simulink model "compare_filters"  (R2025a)
settings: Solver=VariableStepAuto  StartTime=0.0  StopTime=1.5  RelTol=1e-3
values from neighbouring files (symbols this model uses):
  phi_corr_LUT_param = Simulink.Parameter(phi_corr_LUT)    [lut_script.m]
undefined symbols (not defined in the file or in its folder): closed_loop, D_duty_cycle, D_m, DiscIntNeverNeededParam, hall_errors, I_duty_cycle, J_t, L_ss, lambda_m, P, P_duty_cycle, r_s, R_vs, T_m, theta_v, use_LUT, V_bus
libraries: spsMosfetLib x18, spsSeriesRLCBranchLib x12, spsVoltageMeasurementLib x9, spsControlledCurrentSourceLib x9, slpidlib x6, eeGeneralControl x3, simulink x3, embmathops x3, spsControlledVoltageSourceLib x3, spsPWMGeneratorDCDCLib x3, spsDCVoltageSourceLib x3, sps_lib x3
(part 3 of 3)

== system compare_filters/3_phase/hall_filter/hardware_ISR_routine/Subsystem1 ==
  In1 : Inport
  Memory{,1..5} (6 alike) : Memory  InheritSampleTime=on
  Mux : Mux  Inputs=6
  Sum{,1..5} (6 alike) : Sum  Inputs=|+-
  tau_vec : Outport
  wires:
  Memory1/1 -> Sum1/2, Sum2/1, Memory2/1
  Memory/1 -> Sum1/1, Sum/2, Memory1/1
  Memory2/1 -> Sum3/1, Sum2/2, Memory3/1
  In1/1 -> Sum/1, Memory/1
  Memory3/1 -> Sum4/1, Sum3/2, Memory4/1
  Memory4/1 -> Memory5/1, Sum5/1, Sum4/2
  Mux/1 -> tau_vec/1
  Memory5/1 -> Sum5/2
  Sum/1 -> Mux/1
  Sum1/1 -> Mux/2
  Sum2/1 -> Mux/3
  Sum3/1 -> Mux/4
  Sum4/1 -> Mux/5
  Sum5/1 -> Mux/6

== system compare_filters/3_phase/hall_filter/hardware_ISR_routine/Subsystem2 ==
  timer : Inport
  Data Store Write2 : DataStoreWrite  DataStoreName=t_now  IndexOptions=Index vector (dialog)  Indices=1  OutputSizes=1
  wires:
  timer/1 -> Data Store Write2/1

== system compare_filters/3_phase/hall_filter/hardware_ISR_routine/Subsystem3 ==
  tau_now_write : Inport
  tau_next_write : Inport  Port=2
  update_now : Inport  Port=3
  update_next : Inport  Port=4
  Enable : EnablePort
  Subsystem : Subsystem
  Subsystem1 : Subsystem
  wires:
  tau_now_write/1 -> Subsystem/1(tau_now_write)
  tau_next_write/1 -> Subsystem1/1(tau_next_write)
  update_now/1 -> Subsystem/Enable
  update_next/1 -> Subsystem1/Enable

== system compare_filters/3_phase/hall_filter/software_ISR_routine/Subsystem ==
  Data Store Read : DataStoreRead  DataStoreName=tau_corr_next  IndexOptions=Index vector (dialog)  Indices=1  OutputSizes=1
  Data Store Write : DataStoreWrite  DataStoreName=tau_corr_now  IndexOptions=Index vector (dialog)  Indices=1  OutputSizes=1
  wires:
  Data Store Read/1 -> Data Store Write/1

== system compare_filters/3_phase/hall_filter/software_ISR_routine/Subsystem1 ==
  Constant : Constant  Value=-1
  Data Store Write1 : DataStoreWrite  DataStoreName=tau_corr_next  IndexOptions=Index vector (dialog)  Indices=1  OutputSizes=1
  wires:
  Constant/1 -> Data Store Write1/1

== system compare_filters/3_phase/hall_filter/software_ISR_routine/Subsystem2 ==
  Constant : Constant
  Data Store Read : DataStoreRead  DataStoreName=state_out  IndexOptions=Index vector (dialog)  Indices=1  OutputSizes=1
  Data Store Write : DataStoreWrite  DataStoreName=state_out  IndexOptions=Index vector (dialog)  Indices=1  OutputSizes=1
  Modulo by Constant : embmathops/Modulo by Constant  Denominator=6  SimulateUsing=Code generation
  Sum : Sum  Inputs=|++
  wires:
  Constant/1 -> Sum/2
  Data Store Read/1 -> Sum/1
  Sum/1 -> Modulo by Constant/1
  Modulo by Constant/1 -> Data Store Write/1

== system compare_filters/3_phase/hall_filter/software_ISR_routine/Subsystem3 ==
  Constant : Constant
  Data Store Read : DataStoreRead  DataStoreName=state_out  IndexOptions=Index vector (dialog)  Indices=1  OutputSizes=1
  Sum : Sum  Inputs=|++
  state_out : Outport
  wires:
  Data Store Read/1 -> Sum/1
  Sum/1 -> state_out/1
  Constant/1 -> Sum/2

== system compare_filters/3_phase/hall_filter/software_ISR_routine/Subsystem4 ==
  Constant : Constant  Value=0
  Data Store Write : DataStoreWrite  DataStoreName=first_time  IndexOptions=Index vector (dialog)  Indices=1  OutputSizes=1
  wires:
  Constant/1 -> Data Store Write/1

== system compare_filters/from_LUT/hall_filter/calibration_routine/Subsystem ==
  Constant : Constant  Value=pi/3
  Data Store Read : DataStoreRead  DataStoreName=tau_corr_now  IndexOptions=Index vector (dialog)  Indices=1  OutputSizes=1
  Data Store Write : DataStoreWrite  DataStoreName=omega_now  IndexOptions=Index vector (dialog)  Indices=1  OutputSizes=1
  Divide : Product  Inputs=*/
  wires:
  Data Store Read/1 -> Divide/2
  Constant/1 -> Divide/1
  Divide/1 -> Data Store Write/1

== system compare_filters/from_LUT/hall_filter/calibration_routine/Subsystem1 ==
  Data Store Read : DataStoreRead  DataStoreName=tau_corr_now  IndexOptions=Index vector (dialog)  Indices=1  OutputSizes=1
  Data Store Read1 : DataStoreRead  DataStoreName=omega_now  IndexOptions=Index vector (dialog)  Indices=1  OutputSizes=1
  Data Store Write : DataStoreWrite  DataStoreName=del_phi  IndexOptions=Index vector (dialog)  Indices=1  OutputSizes=1
  Product : Product
  wires:
  Data Store Read/1 -> Product/1
  Data Store Read1/1 -> Product/2
  Product/1 -> Data Store Write/1

== system compare_filters/from_LUT/hall_filter/calibration_routine/Subsystem2 ==
  Constant : Constant  Value=6
  Constant1 : Constant  Value=0.02
  Constant2 : Constant  Value=4e-4
  Constant3 : Constant  Value=50
  Data Store Read1 : DataStoreRead  DataStoreName=state_out  IndexOptions=Index vector (dialog)  Indices=1  OutputSizes=1
  Data Store Read2 : DataStoreRead  DataStoreName=del_phi  IndexOptions=Index vector (dialog)  Indices=1  OutputSizes=1
  Data Store Read3 : DataStoreRead  DataStoreName=LUT_phi  IndexOptions=Index vector (dialog)  Indices=1  OutputSizes=1
  Data Store Read4 : DataStoreRead  DataStoreName=LUT_var  IndexOptions=Index vector (dialog)  Indices=1  OutputSizes=1
  Data Store Read5 : DataStoreRead  DataStoreName=LUT_count  IndexOptions=Index vector (dialog)  Indices=1  OutputSizes=1
  Data Store Read6 : DataStoreRead  DataStoreName=LUT_valid  IndexOptions=Index vector (dialog)  Indices=1  OutputSizes=1
  Data Store Read7 : DataStoreRead  DataStoreName=cal_done  IndexOptions=Index vector (dialog)  Indices=1  OutputSizes=1
  Data Store Write : DataStoreWrite  DataStoreName=LUT_phi  IndexOptions=Index vector (dialog)  Indices=1  OutputSizes=1
  Data Store Write1 : DataStoreWrite  DataStoreName=LUT_var  IndexOptions=Index vector (dialog)  Indices=1  OutputSizes=1
  Data Store Write2 : DataStoreWrite  DataStoreName=LUT_count  IndexOptions=Index vector (dialog)  Indices=1  OutputSizes=1
  Data Store Write3 : DataStoreWrite  DataStoreName=LUT_valid  IndexOptions=Index vector (dialog)  Indices=1  OutputSizes=1
  Data Store Write4 : DataStoreWrite  DataStoreName=cal_done  IndexOptions=Index vector (dialog)  Indices=1  OutputSizes=1
  MATLAB Function : MATLAB Function  TreatAsAtomicUnit=on
  wires:
  Data Store Read1/1 -> MATLAB Function/1(k)
  Data Store Read2/1 -> MATLAB Function/2(dphi)
  Data Store Read3/1 -> MATLAB Function/3(phi)
  Data Store Read4/1 -> MATLAB Function/4(varv)
  Data Store Read5/1 -> MATLAB Function/5(cnt)
  Data Store Read6/1 -> MATLAB Function/6(valid)
  Data Store Read7/1 -> MATLAB Function/7(done)
  Constant/1 -> MATLAB Function/8(Nsteady)
  Constant1/1 -> MATLAB Function/9(deadband_rad)
  Constant2/1 -> MATLAB Function/10(var_max)
  Constant3/1 -> MATLAB Function/11(omega_min)
  MATLAB Function/1(phi_n) -> Data Store Write/1
  MATLAB Function/2(varv_n) -> Data Store Write1/1
  MATLAB Function/3(cnt_n) -> Data Store Write2/1
  MATLAB Function/4(valid_n) -> Data Store Write3/1
  MATLAB Function/5(done_n) -> Data Store Write4/1

== system compare_filters/from_LUT/hall_filter/hardware_ISR_routine/Atomic Subsystem ==
  tau_now_write : Inport
  tau_next_write : Inport  Port=2
  update_now : Inport  Port=3
  update_next : Inport  Port=4
  software_ISR_enable : EnablePort
  Subsystem : Subsystem
  Subsystem1 : Subsystem
  wires:
  tau_next_write/1 -> Subsystem1/1(tau_next_write)
  update_now/1 -> Subsystem/Enable
  update_next/1 -> Subsystem1/Enable
  tau_now_write/1 -> Subsystem/1(tau_now_write)

== system compare_filters/from_LUT/hall_filter/hardware_ISR_routine/Subsystem ==
  Constant : Constant
  Data Store Read : DataStoreRead  DataStoreName=reset_toggle  IndexOptions=Index vector (dialog)  Indices=1  OutputSizes=1
  Data Store Read1 : DataStoreRead  DataStoreName=time_base  IndexOptions=Index vector (dialog)  Indices=1  OutputSizes=1
  Data Store Read2 : DataStoreRead  DataStoreName=t_now  IndexOptions=Index vector (dialog)  Indices=1  OutputSizes=1
  Data Store Write : DataStoreWrite  DataStoreName=reset_toggle  IndexOptions=Index vector (dialog)  Indices=1  OutputSizes=1
  Data Store Write1 : DataStoreWrite  DataStoreName=time_base  IndexOptions=Index vector (dialog)  Indices=1  OutputSizes=1
  Sum : Sum  Inputs=|-+
  Sum1 : Sum  Inputs=|++
  wires:
  Sum/1 -> Data Store Write/1  "reset_val"
  Data Store Read/1 -> Sum/1
  Constant/1 -> Sum/2
  Data Store Read1/1 -> Sum1/1
  Sum1/1 -> Data Store Write1/1
  Data Store Read2/1 -> Sum1/2

== system compare_filters/from_LUT/hall_filter/hardware_ISR_routine/Subsystem1 ==
  In1 : Inport
  Memory{,1..5} (6 alike) : Memory  InheritSampleTime=on
  Mux : Mux  Inputs=6
  Sum{,1..5} (6 alike) : Sum  Inputs=|+-
  tau_vec : Outport
  wires:
  Memory1/1 -> Sum1/2, Sum2/1, Memory2/1
  Memory/1 -> Sum1/1, Sum/2, Memory1/1
  Memory2/1 -> Sum3/1, Sum2/2, Memory3/1
  In1/1 -> Sum/1, Memory/1
  Memory3/1 -> Sum4/1, Sum3/2, Memory4/1
  Memory4/1 -> Memory5/1, Sum5/1, Sum4/2
  Mux/1 -> tau_vec/1
  Memory5/1 -> Sum5/2
  Sum/1 -> Mux/1
  Sum1/1 -> Mux/2
  Sum2/1 -> Mux/3
  Sum3/1 -> Mux/4
  Sum4/1 -> Mux/5
  Sum5/1 -> Mux/6

== system compare_filters/from_LUT/hall_filter/hardware_ISR_routine/Subsystem2 ==
  timer : Inport
  Data Store Write2 : DataStoreWrite  DataStoreName=t_now  IndexOptions=Index vector (dialog)  Indices=1  OutputSizes=1
  wires:
  timer/1 -> Data Store Write2/1

== system compare_filters/from_LUT/hall_filter/hardware_ISR_routine/Subsystem3 ==
  tau_now_write : Inport
  tau_next_write : Inport  Port=2
  update_now : Inport  Port=3
  update_next : Inport  Port=4
  Enable : EnablePort
  Subsystem : Subsystem
  Subsystem1 : Subsystem
  wires:
  tau_now_write/1 -> Subsystem/1(tau_now_write)
  tau_next_write/1 -> Subsystem1/1(tau_next_write)
  update_now/1 -> Subsystem/Enable
  update_next/1 -> Subsystem1/Enable

== system compare_filters/from_LUT/hall_filter/software_ISR_routine/Subsystem ==
  Data Store Read : DataStoreRead  DataStoreName=tau_corr_next  IndexOptions=Index vector (dialog)  Indices=1  OutputSizes=1
  Data Store Write : DataStoreWrite  DataStoreName=tau_corr_now  IndexOptions=Index vector (dialog)  Indices=1  OutputSizes=1
  wires:
  Data Store Read/1 -> Data Store Write/1

== system compare_filters/from_LUT/hall_filter/software_ISR_routine/Subsystem1 ==
  Constant : Constant  Value=-1
  Data Store Write1 : DataStoreWrite  DataStoreName=tau_corr_next  IndexOptions=Index vector (dialog)  Indices=1  OutputSizes=1
  wires:
  Constant/1 -> Data Store Write1/1

== system compare_filters/from_LUT/hall_filter/software_ISR_routine/Subsystem2 ==
  Constant : Constant
  Data Store Read : DataStoreRead  DataStoreName=state_out  IndexOptions=Index vector (dialog)  Indices=1  OutputSizes=1
  Data Store Write : DataStoreWrite  DataStoreName=state_out  IndexOptions=Index vector (dialog)  Indices=1  OutputSizes=1
  Modulo by Constant : embmathops/Modulo by Constant  Denominator=6  SimulateUsing=Code generation
  Sum : Sum  Inputs=|++
  wires:
  Constant/1 -> Sum/2
  Data Store Read/1 -> Sum/1
  Sum/1 -> Modulo by Constant/1
  Modulo by Constant/1 -> Data Store Write/1

== system compare_filters/from_LUT/hall_filter/software_ISR_routine/Subsystem3 ==
  Constant : Constant
  Data Store Read : DataStoreRead  DataStoreName=state_out  IndexOptions=Index vector (dialog)  Indices=1  OutputSizes=1
  Sum : Sum  Inputs=|++
  state_out : Outport
  wires:
  Data Store Read/1 -> Sum/1
  Sum/1 -> state_out/1
  Constant/1 -> Sum/2

== system compare_filters/from_LUT/hall_filter/software_ISR_routine/Subsystem4 ==
  Constant : Constant  Value=0
  Data Store Write : DataStoreWrite  DataStoreName=first_time  IndexOptions=Index vector (dialog)  Indices=1  OutputSizes=1
  wires:
  Constant/1 -> Data Store Write/1

== system compare_filters/no_LUT/hall_filter/calibration_routine/Subsystem ==
  Constant : Constant  Value=pi/3
  Data Store Read : DataStoreRead  DataStoreName=tau_corr_now  IndexOptions=Index vector (dialog)  Indices=1  OutputSizes=1
  Data Store Write : DataStoreWrite  DataStoreName=omega_now  IndexOptions=Index vector (dialog)  Indices=1  OutputSizes=1
  Divide : Product  Inputs=*/
  wires:
  Data Store Read/1 -> Divide/2
  Constant/1 -> Divide/1
  Divide/1 -> Data Store Write/1

== system compare_filters/no_LUT/hall_filter/calibration_routine/Subsystem1 ==
  Data Store Read : DataStoreRead  DataStoreName=tau_corr_now  IndexOptions=Index vector (dialog)  Indices=1  OutputSizes=1
  Data Store Read1 : DataStoreRead  DataStoreName=omega_now  IndexOptions=Index vector (dialog)  Indices=1  OutputSizes=1
  Data Store Write : DataStoreWrite  DataStoreName=del_phi  IndexOptions=Index vector (dialog)  Indices=1  OutputSizes=1
  Product : Product
  wires:
  Data Store Read/1 -> Product/1
  Data Store Read1/1 -> Product/2
  Product/1 -> Data Store Write/1

== system compare_filters/no_LUT/hall_filter/calibration_routine/Subsystem2 ==
  Constant : Constant  Value=6
  Constant1 : Constant  Value=0.02
  Constant2 : Constant  Value=4e-4
  Constant3 : Constant  Value=50
  Data Store Read1 : DataStoreRead  DataStoreName=state_out  IndexOptions=Index vector (dialog)  Indices=1  OutputSizes=1
  Data Store Read2 : DataStoreRead  DataStoreName=del_phi  IndexOptions=Index vector (dialog)  Indices=1  OutputSizes=1
  Data Store Read3 : DataStoreRead  DataStoreName=LUT_phi  IndexOptions=Index vector (dialog)  Indices=1  OutputSizes=1
  Data Store Read4 : DataStoreRead  DataStoreName=LUT_var  IndexOptions=Index vector (dialog)  Indices=1  OutputSizes=1
  Data Store Read5 : DataStoreRead  DataStoreName=LUT_count  IndexOptions=Index vector (dialog)  Indices=1  OutputSizes=1
  Data Store Read6 : DataStoreRead  DataStoreName=LUT_valid  IndexOptions=Index vector (dialog)  Indices=1  OutputSizes=1
  Data Store Read7 : DataStoreRead  DataStoreName=cal_done  IndexOptions=Index vector (dialog)  Indices=1  OutputSizes=1
  Data Store Write : DataStoreWrite  DataStoreName=LUT_phi  IndexOptions=Index vector (dialog)  Indices=1  OutputSizes=1
  Data Store Write1 : DataStoreWrite  DataStoreName=LUT_var  IndexOptions=Index vector (dialog)  Indices=1  OutputSizes=1
  Data Store Write2 : DataStoreWrite  DataStoreName=LUT_count  IndexOptions=Index vector (dialog)  Indices=1  OutputSizes=1
  Data Store Write3 : DataStoreWrite  DataStoreName=LUT_valid  IndexOptions=Index vector (dialog)  Indices=1  OutputSizes=1
  Data Store Write4 : DataStoreWrite  DataStoreName=cal_done  IndexOptions=Index vector (dialog)  Indices=1  OutputSizes=1
  MATLAB Function : MATLAB Function  TreatAsAtomicUnit=on
  wires:
  Data Store Read1/1 -> MATLAB Function/1(k)
  Data Store Read2/1 -> MATLAB Function/2(dphi)
  Data Store Read3/1 -> MATLAB Function/3(phi)
  Data Store Read4/1 -> MATLAB Function/4(varv)
  Data Store Read5/1 -> MATLAB Function/5(cnt)
  Data Store Read6/1 -> MATLAB Function/6(valid)
  Data Store Read7/1 -> MATLAB Function/7(done)
  Constant/1 -> MATLAB Function/8(Nsteady)
  Constant1/1 -> MATLAB Function/9(deadband_rad)
  Constant2/1 -> MATLAB Function/10(var_max)
  Constant3/1 -> MATLAB Function/11(omega_min)
  MATLAB Function/1(phi_n) -> Data Store Write/1
  MATLAB Function/2(varv_n) -> Data Store Write1/1
  MATLAB Function/3(cnt_n) -> Data Store Write2/1
  MATLAB Function/4(valid_n) -> Data Store Write3/1
  MATLAB Function/5(done_n) -> Data Store Write4/1

== system compare_filters/no_LUT/hall_filter/hardware_ISR_routine/Atomic Subsystem ==
  tau_now_write : Inport
  tau_next_write : Inport  Port=2
  update_now : Inport  Port=3
  update_next : Inport  Port=4
  software_ISR_enable : EnablePort
  Subsystem : Subsystem
  Subsystem1 : Subsystem
  wires:
  tau_next_write/1 -> Subsystem1/1(tau_next_write)
  update_now/1 -> Subsystem/Enable
  update_next/1 -> Subsystem1/Enable
  tau_now_write/1 -> Subsystem/1(tau_now_write)

== system compare_filters/no_LUT/hall_filter/hardware_ISR_routine/Subsystem ==
  Constant : Constant
  Data Store Read : DataStoreRead  DataStoreName=reset_toggle  IndexOptions=Index vector (dialog)  Indices=1  OutputSizes=1
  Data Store Read1 : DataStoreRead  DataStoreName=time_base  IndexOptions=Index vector (dialog)  Indices=1  OutputSizes=1
  Data Store Read2 : DataStoreRead  DataStoreName=t_now  IndexOptions=Index vector (dialog)  Indices=1  OutputSizes=1
  Data Store Write : DataStoreWrite  DataStoreName=reset_toggle  IndexOptions=Index vector (dialog)  Indices=1  OutputSizes=1
  Data Store Write1 : DataStoreWrite  DataStoreName=time_base  IndexOptions=Index vector (dialog)  Indices=1  OutputSizes=1
  Sum : Sum  Inputs=|-+
  Sum1 : Sum  Inputs=|++
  wires:
  Sum/1 -> Data Store Write/1  "reset_val"
  Data Store Read/1 -> Sum/1
  Constant/1 -> Sum/2
  Data Store Read1/1 -> Sum1/1
  Sum1/1 -> Data Store Write1/1
  Data Store Read2/1 -> Sum1/2

== system compare_filters/no_LUT/hall_filter/hardware_ISR_routine/Subsystem1 ==
  In1 : Inport
  Memory{,1..5} (6 alike) : Memory  InheritSampleTime=on
  Mux : Mux  Inputs=6
  Sum{,1..5} (6 alike) : Sum  Inputs=|+-
  tau_vec : Outport
  wires:
  Memory1/1 -> Sum1/2, Sum2/1, Memory2/1
  Memory/1 -> Sum1/1, Sum/2, Memory1/1
  Memory2/1 -> Sum3/1, Sum2/2, Memory3/1
  In1/1 -> Sum/1, Memory/1
  Memory3/1 -> Sum4/1, Sum3/2, Memory4/1
  Memory4/1 -> Memory5/1, Sum5/1, Sum4/2
  Mux/1 -> tau_vec/1
  Memory5/1 -> Sum5/2
  Sum/1 -> Mux/1
  Sum1/1 -> Mux/2
  Sum2/1 -> Mux/3
  Sum3/1 -> Mux/4
  Sum4/1 -> Mux/5
  Sum5/1 -> Mux/6

== system compare_filters/no_LUT/hall_filter/hardware_ISR_routine/Subsystem2 ==
  timer : Inport
  Data Store Write2 : DataStoreWrite  DataStoreName=t_now  IndexOptions=Index vector (dialog)  Indices=1  OutputSizes=1
  wires:
  timer/1 -> Data Store Write2/1

== system compare_filters/no_LUT/hall_filter/hardware_ISR_routine/Subsystem3 ==
  tau_now_write : Inport
  tau_next_write : Inport  Port=2
  update_now : Inport  Port=3
  update_next : Inport  Port=4
  Enable : EnablePort
  Subsystem : Subsystem
  Subsystem1 : Subsystem
  wires:
  tau_now_write/1 -> Subsystem/1(tau_now_write)
  tau_next_write/1 -> Subsystem1/1(tau_next_write)
  update_now/1 -> Subsystem/Enable
  update_next/1 -> Subsystem1/Enable

== system compare_filters/no_LUT/hall_filter/software_ISR_routine/Subsystem ==
  Data Store Read : DataStoreRead  DataStoreName=tau_corr_next  IndexOptions=Index vector (dialog)  Indices=1  OutputSizes=1
  Data Store Write : DataStoreWrite  DataStoreName=tau_corr_now  IndexOptions=Index vector (dialog)  Indices=1  OutputSizes=1
  wires:
  Data Store Read/1 -> Data Store Write/1

== system compare_filters/no_LUT/hall_filter/software_ISR_routine/Subsystem1 ==
  Constant : Constant  Value=-1
  Data Store Write1 : DataStoreWrite  DataStoreName=tau_corr_next  IndexOptions=Index vector (dialog)  Indices=1  OutputSizes=1
  wires:
  Constant/1 -> Data Store Write1/1

== system compare_filters/no_LUT/hall_filter/software_ISR_routine/Subsystem2 ==
  Constant : Constant
  Data Store Read : DataStoreRead  DataStoreName=state_out  IndexOptions=Index vector (dialog)  Indices=1  OutputSizes=1
  Data Store Write : DataStoreWrite  DataStoreName=state_out  IndexOptions=Index vector (dialog)  Indices=1  OutputSizes=1
  Modulo by Constant : embmathops/Modulo by Constant  Denominator=6  SimulateUsing=Code generation
  Sum : Sum  Inputs=|++
  wires:
  Constant/1 -> Sum/2
  Data Store Read/1 -> Sum/1
  Sum/1 -> Modulo by Constant/1
  Modulo by Constant/1 -> Data Store Write/1

== system compare_filters/no_LUT/hall_filter/software_ISR_routine/Subsystem3 ==
  Constant : Constant
  Data Store Read : DataStoreRead  DataStoreName=state_out  IndexOptions=Index vector (dialog)  Indices=1  OutputSizes=1
  Sum : Sum  Inputs=|++
  state_out : Outport
  wires:
  Data Store Read/1 -> Sum/1
  Sum/1 -> state_out/1
  Constant/1 -> Sum/2

== system compare_filters/no_LUT/hall_filter/software_ISR_routine/Subsystem4 ==
  Constant : Constant  Value=0
  Data Store Write : DataStoreWrite  DataStoreName=first_time  IndexOptions=Index vector (dialog)  Indices=1  OutputSizes=1
  wires:
  Constant/1 -> Data Store Write/1

== system compare_filters/3_phase/hall_filter/hardware_ISR_routine/Atomic Subsystem/Subsystem ==
  tau_now_write : Inport
  update_now : EnablePort
  Data Store Write : DataStoreWrite  DataStoreName=tau_corr_now  IndexOptions=Index vector (dialog)  Indices=1  OutputSizes=1
  wires:
  tau_now_write/1 -> Data Store Write/1

== system compare_filters/3_phase/hall_filter/hardware_ISR_routine/Atomic Subsystem/Subsystem1 ==
  tau_next_write : Inport
  update_next : EnablePort
  Data Store Write1 : DataStoreWrite  DataStoreName=tau_corr_next  IndexOptions=Index vector (dialog)  Indices=1  OutputSizes=1
  wires:
  tau_next_write/1 -> Data Store Write1/1

== system compare_filters/3_phase/hall_filter/hardware_ISR_routine/Subsystem3/Subsystem ==
  tau_now_write : Inport
  update_now : EnablePort
  Data Store Write : DataStoreWrite  DataStoreName=tau_corr_now  IndexOptions=Index vector (dialog)  Indices=1  OutputSizes=1
  wires:
  tau_now_write/1 -> Data Store Write/1

== system compare_filters/3_phase/hall_filter/hardware_ISR_routine/Subsystem3/Subsystem1 ==
  tau_next_write : Inport
  update_next : EnablePort
  Data Store Write1 : DataStoreWrite  DataStoreName=tau_corr_next  IndexOptions=Index vector (dialog)  Indices=1  OutputSizes=1
  wires:
  tau_next_write/1 -> Data Store Write1/1

== system compare_filters/from_LUT/hall_filter/hardware_ISR_routine/Atomic Subsystem/Subsystem ==
  tau_now_write : Inport
  update_now : EnablePort
  Data Store Write : DataStoreWrite  DataStoreName=tau_corr_now  IndexOptions=Index vector (dialog)  Indices=1  OutputSizes=1
  wires:
  tau_now_write/1 -> Data Store Write/1

== system compare_filters/from_LUT/hall_filter/hardware_ISR_routine/Atomic Subsystem/Subsystem1 ==
  tau_next_write : Inport
  update_next : EnablePort
  Data Store Write1 : DataStoreWrite  DataStoreName=tau_corr_next  IndexOptions=Index vector (dialog)  Indices=1  OutputSizes=1
  wires:
  tau_next_write/1 -> Data Store Write1/1

== system compare_filters/from_LUT/hall_filter/hardware_ISR_routine/Subsystem3/Subsystem ==
  tau_now_write : Inport
  update_now : EnablePort
  Data Store Write : DataStoreWrite  DataStoreName=tau_corr_now  IndexOptions=Index vector (dialog)  Indices=1  OutputSizes=1
  wires:
  tau_now_write/1 -> Data Store Write/1

== system compare_filters/from_LUT/hall_filter/hardware_ISR_routine/Subsystem3/Subsystem1 ==
  tau_next_write : Inport
  update_next : EnablePort
  Data Store Write1 : DataStoreWrite  DataStoreName=tau_corr_next  IndexOptions=Index vector (dialog)  Indices=1  OutputSizes=1
  wires:
  tau_next_write/1 -> Data Store Write1/1

== system compare_filters/no_LUT/hall_filter/hardware_ISR_routine/Atomic Subsystem/Subsystem ==
  tau_now_write : Inport
  update_now : EnablePort
  Data Store Write : DataStoreWrite  DataStoreName=tau_corr_now  IndexOptions=Index vector (dialog)  Indices=1  OutputSizes=1
  wires:
  tau_now_write/1 -> Data Store Write/1

== system compare_filters/no_LUT/hall_filter/hardware_ISR_routine/Atomic Subsystem/Subsystem1 ==
  tau_next_write : Inport
  update_next : EnablePort
  Data Store Write1 : DataStoreWrite  DataStoreName=tau_corr_next  IndexOptions=Index vector (dialog)  Indices=1  OutputSizes=1
  wires:
  tau_next_write/1 -> Data Store Write1/1

== system compare_filters/no_LUT/hall_filter/hardware_ISR_routine/Subsystem3/Subsystem ==
  tau_now_write : Inport
  update_now : EnablePort
  Data Store Write : DataStoreWrite  DataStoreName=tau_corr_now  IndexOptions=Index vector (dialog)  Indices=1  OutputSizes=1
  wires:
  tau_now_write/1 -> Data Store Write/1

== system compare_filters/no_LUT/hall_filter/hardware_ISR_routine/Subsystem3/Subsystem1 ==
  tau_next_write : Inport
  update_next : EnablePort
  Data Store Write1 : DataStoreWrite  DataStoreName=tau_corr_next  IndexOptions=Index vector (dialog)  Indices=1  OutputSizes=1
  wires:
  tau_next_write/1 -> Data Store Write1/1

== matlab function compare_filters/from_LUT/hall_filter/MATLAB Function1 ==
  data: interval input; num output
function num = interval_to_num(interval)
DICT = [4,6,2,3,1,5];
if interval == 0
    num = 0;
else
    num = DICT(interval);
end

== matlab function compare_filters/from_LUT/hall_filter/hardware_ISR_routine/MATLAB Function ==
  data: timer input; tau_now_out output; tau_vec input; tau_now input; tau_next input; tau_next_out output; update_now output; update_next output; tau_corr_out output; tau_LUT_input input; use_LUT input; state_out input
function [tau_now_out, tau_next_out, update_now, update_next, tau_corr_out] = ...
    update_tau_vals_conditional(timer, tau_vec, tau_now, tau_next, ...
                                tau_LUT_input, use_LUT, state_out)

    % 0. Software sector index (0..5)
    persistent sector_idx
    if isempty(sector_idx)
        % Optionally use state_out at startup so you're aligned
        sector_idx = uint8(mod(state_out, 6));  % 0..5
    end

    % 1. Initialize outputs
    tau_now_out  = 0.0;
    tau_next_out = 0.0;
    tau_corr     = 0.0;

    % 2. Compute tau_corr from filter or LUT
    if use_LUT == 1
        % --- LUT MODE: ignore live state_out, use software sector index ---
        tau_corr = tau_LUT_input(sector_idx + 1);   % sector_idx = 0..5
    else
        % --- Quadratic Filter ---
        % tau_corr = (1/3) * ( 4*tau_vec(1) ...
        %                    -    tau_vec(2) ...
        %                    + 2*tau_vec(3) ...
        %                    - 4*tau_vec(4) ...
        %                    + 2*tau_vec(5));

        % --- Six Step Filter ---
        tau_corr = 1/3 * (-tau_vec(1)+tau_vec(3)+tau_vec(4)+tau_vec(5)+tau_vec(6));
    end

    tau_corr_out = tau_corr;

    % 3. Schedule interrupts (unchanged)
    update_now  = false;
    update_next = false;

    if timer <= tau_now
        tau_now_out  = tau_now;          % keep current
        tau_next_out = timer + tau_corr; % schedule next
        update_next  = true;
    else
        tau_now_out  = timer + tau_corr; % schedule now
        tau_next_out = tau_next;         % keep next
        update_now   = true;
    end

    % 4. Advance software sector index once per commutation
    % This function is called once per commutation event, so just walk 0..5.
    if use_LUT == 1
        sector_idx = uint8(mod(double(sector_idx) + 1, 6));
    else
        % In calibration mode you *can* still use state_out if you want to
        % write back into the LUT elsewhere, but here we just leave
        % sector_idx alone or optionally keep it synced:
        % sector_idx = uint8(mod(state_out, 6));
    end
end

== matlab function compare_filters/no_LUT/MATLAB Function1 ==
  data: omega_r input; f_Hz output
function f_Hz = avg_freq_sim(omega_r)
f_Hz = avg_freq(omega_r);

== matlab function compare_filters/from_LUT/hall_filter/calibration_routine/Subsystem2/MATLAB Function ==
  data: k input; phi_n output; dphi input; phi input; varv input; cnt input; valid input; done input; Nsteady input; deadband_rad input; var_max input; omega_min input; varv_n output; cnt_n output; valid_n output; done_n output
function [phi_n,varv_n,cnt_n,valid_n,done_n] = lut_update_one( ...
    k, dphi, phi, varv, cnt, valid, done, ...
    Nsteady, deadband_rad, var_max, omega_min)

% Copy-through defaults
phi_n   = phi;
varv_n  = varv;
cnt_n   = cnt;
valid_n = valid;
done_n  = done;

% Guard: out-of-range index or already done
if done || k < 1 || k > 6
    return;
end

% ---- Welford mean/variance update for entry k ----
n  = double(cnt(k));
mu = double(phi(k));
M2 = double(varv(k)) * max(n - 1, 0);

n  = n + 1;
if n == 1
    mu = double(dphi);
    M2 = 0.0;
else
    delta = double(dphi) - mu;
    mu    = mu + delta / n;
    M2    = M2 + delta * (double(dphi) - mu);
end

cnt_n(k)  = uint8(min(n, 255));
phi_n(k)  = single(mu);
if n > 1
    varv_n(k) = single(M2 / (n - 1));
else
    varv_n(k) = single(0);
end

% ---- Validity for this state ----
close_ok = (abs(double(dphi) - mu) <= double(deadband_rad));
var_ok   = (double(varv_n(k))      <= double(var_max));
count_ok = (n >= double(Nsteady));
if close_ok && var_ok && count_ok
    valid_n(k) = true;
end

% ---- Global done ----
allv = true;
for i = 1:6
    allv = allv && valid_n(i);
end
if allv
    done_n = true;
end

== matlab function compare_filters/from_LUT/hall_filter/hardware_ISR_routine/MATLAB Function1 ==
  data: tau_LUT_input input; tau_corr_LUT_test output
function tau_corr_LUT_test = tau_corr_LUT_test_fn(tau_LUT_input)
%#codegen
% tau_LUT_input : 6x1 or 1x6 vector of tau values for sectors 0..5
% use_LUT       : scalar flag (0/1), lets you freeze counter in filter mode

    % Software sector index (0..5), independent of Hall state
    persistent sector_idx
    if isempty(sector_idx)
        sector_idx = uint8(0);  % internal counter 0..5
    end

    % --- sector phase offset in "steps" (−1 step == +5 mod 6) ---
    % Adjust this if you find it leads instead of lags.
    offset = int8(-1);    % one-sector *earlier* than the counter
    % offset = +1 would be one-sector later, etc.

    % Default output
    tau_corr_LUT_test = 0.0;

    % Compute current LUT index with phase offset
    k = int8(sector_idx) + offset;       % may be negative
    k = mod(double(k), 6);               % wrap into 0..5
    idx = uint8(k) + 1;                  % 1-based for MATLAB

    % Use LUT entry
    tau_corr_LUT_test = tau_LUT_input(idx);

    % Only advance the counter when LUT mode is active

        sector_idx = uint8(mod(double(sector_idx) + 1, 6));
    
end

== matlab function compare_filters/no_LUT/controller_1 ==
  data: HALL_STATE input; T_vec output
function T_vec = controller_6step_120_sim(HALL_STATE)
T_vec = controller_6step_120(HALL_STATE);
end

== matlab function compare_filters/no_LUT/hall sensors ==
  data: hall_errors input; theta_r input; H1 output; H2 output; H3 output
function [H1,H2,H3] = hall_sensor_sim(hall_errors, theta_r)
[H1,H2,H3] = hall_sensor(theta_r, hall_errors);
end

== matlab function compare_filters/no_LUT/hall_filter/First trigger initialization/MATLAB Function ==
  data: num input; interval output
function interval = num_to_interval(num)
DICT = [5,3,4,1,6,2];
interval = DICT(num);

== matlab function compare_filters/no_LUT/hall_filter/MATLAB Function ==
  data: H1 input; HALL_STATE output; H2 input; H3 input
function HALL_STATE = hall_to_statenum(H1,H2,H3)
HALL_STATE = 4*H1 + 2*H2 + H3;

== matlab function compare_filters/no_LUT/hall_filter/MATLAB Function1 ==
  data: interval input; num output
function num = interval_to_num(interval)
DICT = [4,6,2,3,1,5];
if interval == 0
    num = 0;
else
    num = DICT(interval);
end

== matlab function compare_filters/no_LUT/hall_filter/calibration_routine/Subsystem2/MATLAB Function ==
  data: k input; phi_n output; dphi input; phi input; varv input; cnt input; valid input; done input; Nsteady input; deadband_rad input; var_max input; omega_min input; varv_n output; cnt_n output; valid_n output; done_n output
function [phi_n,varv_n,cnt_n,valid_n,done_n] = lut_update_one( ...
    k, dphi, phi, varv, cnt, valid, done, ...
    Nsteady, deadband_rad, var_max, omega_min)

% Copy-through defaults
phi_n   = phi;
varv_n  = varv;
cnt_n   = cnt;
valid_n = valid;
done_n  = done;

% Guard: out-of-range index or already done
if done || k < 1 || k > 6
    return;
end

% ---- Welford mean/variance update for entry k ----
n  = double(cnt(k));
mu = double(phi(k));
M2 = double(varv(k)) * max(n - 1, 0);

n  = n + 1;
if n == 1
    mu = double(dphi);
    M2 = 0.0;
else
    delta = double(dphi) - mu;
    mu    = mu + delta / n;
    M2    = M2 + delta * (double(dphi) - mu);
end

cnt_n(k)  = uint8(min(n, 255));
phi_n(k)  = single(mu);
if n > 1
    varv_n(k) = single(M2 / (n - 1));
else
    varv_n(k) = single(0);
end

% ---- Validity for this state ----
close_ok = (abs(double(dphi) - mu) <= double(deadband_rad));
var_ok   = (double(varv_n(k))      <= double(var_max));
count_ok = (n >= double(Nsteady));
if close_ok && var_ok && count_ok
    valid_n(k) = true;
end

% ---- Global done ----
allv = true;
for i = 1:6
    allv = allv && valid_n(i);
end
if allv
    done_n = true;
end

== matlab function compare_filters/from_LUT/qd-frame to stator ==
  data: fa output; fb output; fc output; fq input; fd input; theta input
function [fa,fb,fc] = K_mat_inv_sim(fq,fd,theta)
[fa,fb,fc] = K_mat_inv(fq,fd,theta);

== matlab function compare_filters/no_LUT/hall_filter/hardware_ISR_routine/MATLAB Function ==
  data: timer input; tau_now_out output; tau_vec input; tau_now input; tau_next input; tau_next_out output; update_now output; update_next output; tau_corr_out output; tau_LUT_input input; use_LUT input; state_out input
function [tau_now_out, tau_next_out, update_now, update_next, tau_corr_out] = ...
    update_tau_vals_conditional(timer, tau_vec, tau_now, tau_next, ...
                                tau_LUT_input, use_LUT, state_out)

    % 0. Software sector index (0..5)
    persistent sector_idx
    if isempty(sector_idx)
        % Optionally use state_out at startup so you're aligned
        sector_idx = uint8(mod(state_out, 6));  % 0..5
    end

    % 1. Initialize outputs
    tau_now_out  = 0.0;
    tau_next_out = 0.0;
    tau_corr     = 0.0;

    use_LUT;

    % % 2. Compute tau_corr from filter or LUT
    % if use_LUT == 1
    %     % --- LUT MODE: ignore live state_out, use software sector index ---
    %     tau_corr = tau_LUT_input(sector_idx + 1);   % sector_idx = 0..5
    % else
        % --- Quadratic Filter ---
        % tau_corr = (1/3) * ( 4*tau_vec(1) ...
        %                    -    tau_vec(2) ...
        %                    + 2*tau_vec(3) ...
        %                    - 4*tau_vec(4) ...
        %                    + 2*tau_vec(5));
        % --- Six Step Filter ---
        tau_corr = 1/3 * (-tau_vec(1)+tau_vec(3)+tau_vec(4)+tau_vec(5)+tau_vec(6));
    % end

    tau_corr_out = tau_corr;

    % 3. Schedule interrupts (unchanged)
    update_now  = false;
    update_next = false;

    if timer <= tau_now
        tau_now_out  = tau_now;          % keep current
        tau_next_out = timer + tau_corr; % schedule next
        update_next  = true;
    else
        tau_now_out  = timer + tau_corr; % schedule now
        tau_next_out = tau_next;         % keep next
        update_now   = true;
    end

    % 4. Advance software sector index once per commutation
    % This function is called once per commutation event, so just walk 0..5.
    if use_LUT == 1
        sector_idx = uint8(mod(double(sector_idx) + 1, 6));
    else
        % In calibration mode you *can* still use state_out if you want to
        % write back into the LUT elsewhere, but here we just leave
        % sector_idx alone or optionally keep it synced:
        % sector_idx = uint8(mod(state_out, 6));
    end
end

== matlab function compare_filters/no_LUT/hall_filter/hardware_ISR_routine/MATLAB Function1 ==
  data: tau_LUT_input input; tau_corr_LUT_test output
function tau_corr_LUT_test = tau_corr_LUT_test_fn(tau_LUT_input)
%#codegen
% tau_LUT_input : 6x1 or 1x6 vector of tau values for sectors 0..5
% use_LUT       : scalar flag (0/1), lets you freeze counter in filter mode

    % Software sector index (0..5), independent of Hall state
    persistent sector_idx
    if isempty(sector_idx)
        sector_idx = uint8(0);  % internal counter 0..5
    end

    % --- sector phase offset in "steps" (−1 step == +5 mod 6) ---
    % Adjust this if you find it leads instead of lags.
    offset = int8(-1);    % one-sector *earlier* than the counter
    % offset = +1 would be one-sector later, etc.

    % Default output
    tau_corr_LUT_test = 0.0;

    % Compute current LUT index with phase offset
    k = int8(sector_idx) + offset;       % may be negative
    k = mod(double(k), 6);               % wrap into 0..5
    idx = uint8(k) + 1;                  % 1-based for MATLAB

    % Use LUT entry
    tau_corr_LUT_test = tau_LUT_input(idx);

    % Only advance the counter when LUT mode is active

        sector_idx = uint8(mod(double(sector_idx) + 1, 6));
    
end

== matlab function compare_filters/no_LUT/qd-frame to stator ==
  data: fa output; fb output; fc output; fq input; fd input; theta input
function [fa,fb,fc] = K_mat_inv_sim(fq,fd,theta)
[fa,fb,fc] = K_mat_inv(fq,fd,theta);

== matlab function compare_filters/no_LUT/stator to qd-frame ==
  data: fa input; fq output; fb input; fc input; theta input; fd output
function [fq,fd] = K_mat_sim(fa,fb,fc,theta)
[fq,fd] = K_mat(fa,fb,fc,theta);

== matlab function compare_filters/3_phase/MATLAB Function ==
  data: H1 input; HALL_STATE output; H2 input; H3 input
function HALL_STATE = hall_to_statenum(H1,H2,H3)
HALL_STATE = 4*H1 + 2*H2 + H3;

== matlab function compare_filters/3_phase/MATLAB Function1 ==
  data: omega_r input; f_Hz output
function f_Hz = avg_freq_sim(omega_r)
f_Hz = avg_freq(omega_r);

== matlab function compare_filters/3_phase/controller_1 ==
  data: HALL_STATE input; T_vec output
function T_vec = controller_6step_120_sim(HALL_STATE)
T_vec = controller_6step_120(HALL_STATE);
end

== matlab function compare_filters/3_phase/hall sensors ==
  data: hall_errors input; theta_r input; H1 output; H2 output; H3 output
function [H1,H2,H3] = hall_sensor_sim(hall_errors, theta_r)
[H1,H2,H3] = hall_sensor(theta_r, hall_errors);
end

== matlab function compare_filters/3_phase/hall_filter/First trigger initialization/MATLAB Function ==
  data: num input; interval output
function interval = num_to_interval(num)
DICT = [5,3,4,1,6,2];
interval = DICT(num);

== matlab function compare_filters/3_phase/hall_filter/MATLAB Function ==
  data: H1 input; HALL_STATE output; H2 input; H3 input
function HALL_STATE = hall_to_statenum(H1,H2,H3)
HALL_STATE = 4*H1 + 2*H2 + H3;

== matlab function compare_filters/3_phase/hall_filter/MATLAB Function1 ==
  data: interval input; num output
function num = interval_to_num(interval)
DICT = [4,6,2,3,1,5];
if interval == 0
    num = 0;
else
    num = DICT(interval);
end

== matlab function compare_filters/from_LUT/stator to qd-frame ==
  data: fa input; fq output; fb input; fc input; theta input; fd output
function [fq,fd] = K_mat_sim(fa,fb,fc,theta)
[fq,fd] = K_mat(fa,fb,fc,theta);

== matlab function compare_filters/3_phase/hall_filter/calibration_routine/Subsystem2/MATLAB Function ==
  data: k input; phi_n output; dphi input; phi input; varv input; cnt input; valid input; done input; Nsteady input; deadband_rad input; var_max input; omega_min input; varv_n output; cnt_n output; valid_n output; done_n output
function [phi_n,varv_n,cnt_n,valid_n,done_n] = lut_update_one( ...
    k, dphi, phi, varv, cnt, valid, done, ...
    Nsteady, deadband_rad, var_max, omega_min)

% Copy-through defaults
phi_n   = phi;
varv_n  = varv;
cnt_n   = cnt;
valid_n = valid;
done_n  = done;

% Guard: out-of-range index or already done
if done || k < 1 || k > 6
    return;
end

% ---- Welford mean/variance update for entry k ----
n  = double(cnt(k));
mu = double(phi(k));
M2 = double(varv(k)) * max(n - 1, 0);

n  = n + 1;
if n == 1
    mu = double(dphi);
    M2 = 0.0;
else
    delta = double(dphi) - mu;
    mu    = mu + delta / n;
    M2    = M2 + delta * (double(dphi) - mu);
end

cnt_n(k)  = uint8(min(n, 255));
phi_n(k)  = single(mu);
if n > 1
    varv_n(k) = single(M2 / (n - 1));
else
    varv_n(k) = single(0);
end

% ---- Validity for this state ----
close_ok = (abs(double(dphi) - mu) <= double(deadband_rad));
var_ok   = (double(varv_n(k))      <= double(var_max));
count_ok = (n >= double(Nsteady));
if close_ok && var_ok && count_ok
    valid_n(k) = true;
end

% ---- Global done ----
allv = true;
for i = 1:6
    allv = allv && valid_n(i);
end
if allv
    done_n = true;
end

== matlab function compare_filters/3_phase/hall_filter/hardware_ISR_routine/MATLAB Function ==
  data: timer input; tau_now_out output; tau_vec input; tau_now input; tau_next input; tau_next_out output; update_now output; update_next output; tau_corr_out output; tau_LUT_input input; use_LUT input; state_out input
function [tau_now_out, tau_next_out, update_now, update_next, tau_corr_out] = ...
    update_tau_vals_conditional(timer, tau_vec, tau_now, tau_next, ...
                                tau_LUT_input, use_LUT, state_out)

    % 0. Software sector index (0..5)
    persistent sector_idx
    if isempty(sector_idx)
        % Optionally use state_out at startup so you're aligned
        sector_idx = uint8(mod(state_out, 6));  % 0..5
    end

    % 1. Initialize outputs
    tau_now_out  = 0.0;
    tau_next_out = 0.0;
    tau_corr     = 0.0;

    use_LUT;

    % % 2. Compute tau_corr from filter or LUT
    % if use_LUT == 1
    %     % --- LUT MODE: ignore live state_out, use software sector index ---
    %     tau_corr = tau_LUT_input(sector_idx + 1);   % sector_idx = 0..5
    % else
        % --- Quadratic Filter ---
        % tau_corr = (1/3) * ( 4*tau_vec(1) ...
        %                    -    tau_vec(2) ...
        %                    + 2*tau_vec(3) ...
        %                    - 4*tau_vec(4) ...
        %                    + 2*tau_vec(5));
        % % --- Six Step Filter ---
        % tau_corr = 1/3 * (-tau_vec(1)+tau_vec(3)+tau_vec(4)+tau_vec(5)+tau_vec(6));

        % --- Three Step Filter ---
        tau_corr = 1/3 * (tau_vec(2)+2*tau_vec(3));

    % end

    tau_corr_out = tau_corr;

    % 3. Schedule interrupts (unchanged)
    update_now  = false;
    update_next = false;

    if timer <= tau_now
        tau_now_out  = tau_now;          % keep current
        tau_next_out = timer + tau_corr; % schedule next
        update_next  = true;
    else
        tau_now_out  = timer + tau_corr; % schedule now
        tau_next_out = tau_next;         % keep next
        update_now   = true;
    end

    % 4. Advance software sector index once per commutation
    % This function is called once per commutation event, so just walk 0..5.
    if use_LUT == 1
        sector_idx = uint8(mod(double(sector_idx) + 1, 6));
    else
        % In calibration mode you *can* still use state_out if you want to
        % write back into the LUT elsewhere, but here we just leave
        % sector_idx alone or optionally keep it synced:
        % sector_idx = uint8(mod(state_out, 6));
    end
end

== matlab function compare_filters/3_phase/hall_filter/hardware_ISR_routine/MATLAB Function1 ==
  data: tau_LUT_input input; tau_corr_LUT_test output
function tau_corr_LUT_test = tau_corr_LUT_test_fn(tau_LUT_input)
%#codegen
% tau_LUT_input : 6x1 or 1x6 vector of tau values for sectors 0..5
% use_LUT       : scalar flag (0/1), lets you freeze counter in filter mode

    % Software sector index (0..5), independent of Hall state
    persistent sector_idx
    if isempty(sector_idx)
        sector_idx = uint8(0);  % internal counter 0..5
    end

    % --- sector phase offset in "steps" (−1 step == +5 mod 6) ---
    % Adjust this if you find it leads instead of lags.
    offset = int8(-1);    % one-sector *earlier* than the counter
    % offset = +1 would be one-sector later, etc.

    % Default output
    tau_corr_LUT_test = 0.0;

    % Compute current LUT index with phase offset
    k = int8(sector_idx) + offset;       % may be negative
    k = mod(double(k), 6);               % wrap into 0..5
    idx = uint8(k) + 1;                  % 1-based for MATLAB

    % Use LUT entry
    tau_corr_LUT_test = tau_LUT_input(idx);

    % Only advance the counter when LUT mode is active

        sector_idx = uint8(mod(double(sector_idx) + 1, 6));
    
end

== matlab function compare_filters/3_phase/qd-frame to stator ==
  data: fa output; fb output; fc output; fq input; fd input; theta input
function [fa,fb,fc] = K_mat_inv_sim(fq,fd,theta)
[fa,fb,fc] = K_mat_inv(fq,fd,theta);

== matlab function compare_filters/3_phase/stator to qd-frame ==
  data: fa input; fq output; fb input; fc input; theta input; fd output
function [fq,fd] = K_mat_sim(fa,fb,fc,theta)
[fq,fd] = K_mat(fa,fb,fc,theta);

== matlab function compare_filters/from_LUT/controller_1 ==
  data: HALL_STATE input; T_vec output
function T_vec = controller_6step_120_sim(HALL_STATE)
T_vec = controller_6step_120(HALL_STATE);
end

== matlab function compare_filters/from_LUT/hall sensors ==
  data: hall_errors input; theta_r input; H1 output; H2 output; H3 output
function [H1,H2,H3] = hall_sensor_sim(hall_errors, theta_r)
[H1,H2,H3] = hall_sensor(theta_r, hall_errors);
end

== matlab function compare_filters/no_LUT/MATLAB Function ==
  data: H1 input; HALL_STATE output; H2 input; H3 input
function HALL_STATE = hall_to_statenum(H1,H2,H3)
HALL_STATE = 4*H1 + 2*H2 + H3;

== matlab function compare_filters/from_LUT/MATLAB Function ==
  data: H1 input; HALL_STATE output; H2 input; H3 input
function HALL_STATE = hall_to_statenum(H1,H2,H3)
HALL_STATE = 4*H1 + 2*H2 + H3;

== matlab function compare_filters/from_LUT/hall_filter/First trigger initialization/MATLAB Function ==
  data: num input; interval output
function interval = num_to_interval(num)
DICT = [5,3,4,1,6,2];
interval = DICT(num);

== matlab function compare_filters/from_LUT/MATLAB Function1 ==
  data: omega_r input; f_Hz output
function f_Hz = avg_freq_sim(omega_r)
f_Hz = avg_freq(omega_r);

== matlab function compare_filters/from_LUT/hall_filter/MATLAB Function ==
  data: H1 input; HALL_STATE output; H2 input; H3 input
function HALL_STATE = hall_to_statenum(H1,H2,H3)
HALL_STATE = 4*H1 + 2*H2 + H3;
